simulink model "Full H-bridge motor driver simulator"  (R2018a)
settings: Solver=VariableStepAuto  StartTime=0.0  StopTime=20  RelTol=1e-3
undefined symbols (not defined in the file or in its folder): sigbuilder_block
libraries: fl_lib x12, nesl_utility x6, powerlib_meascontrol x1
settings Model: Creator=Kalindi  LastModifiedBy=Kalindi

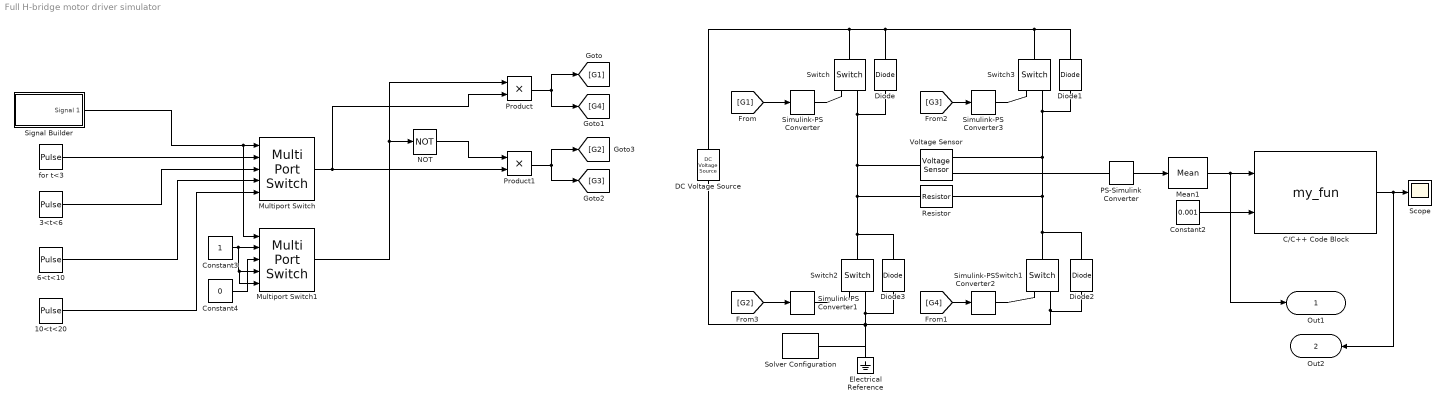
== system Full H-bridge motor driver simulator ==
  10<t<20 : DiscretePulseGenerator  PulseType=Time based  Amplitude=10  Period=0.03125  PulseWidth=79.392
  3<t<6 : DiscretePulseGenerator  PulseType=Time based  Amplitude=10  Period=0.03125  PulseWidth=49.386
  6<t<10 : DiscretePulseGenerator  PulseType=Time based  Amplitude=10  Period=0.03125  PulseWidth=19.956
  C/C++ Code Block : S-Function  InitFcn=try, set_param(gcb,'FunctionName','my_fun'), end  FunctionName=my_fun  Parameters=4.67,0.3234,0.4953  SFunctionModules=my_fun_wrapper  SFunctionDeploymentMode=off  EnableBusSupport=off  mask(S-Function Builder){R=0}
      mask help: Simulink:masks:SFunctionBuilder_MD
      mask init:
      | val = [[.9  0.75 0.75 1 1 .9 .9 1]',[1 1 0.75 0.75 .9 .9 1 .9]'];try , sys = get_param(gcb,'SfunBuilderFcnName');if isempty(sys), sys = get_param(gcb,'FunctionName'); end,catch, sys = get_param(gcb,'FunctionName'); end
      settings: CopyFcn=set_param(gcbh,'LinkStatus','none')  PreSaveFcn=try, set_param(gcb,'FunctionName','my_fun'), end  OpenFcn=sfunctionwizard(gcbh)
      mask Display: plot(val(:,1),val(:,2)),disp(sys), port_label('input',1,'Voltage'), port_label('input',2,'Torque'), port_label('output',1,'Speed')
  Constant2 : Constant  Value=0.001
  Constant3 : Constant
  Constant4 : Constant  Value=0
  DC Voltage Source : fl_lib/Electrical/Electrical Sources/DC Voltage Source  v0=10 V
  Diode{,1..3} (4 alike) : fl_lib/Electrical/Electrical Elements/Diode  Vf=0.6 V  Ron=0.3 Ohm  Goff=1e-8 1/Ohm  i_specify=off  i_priority=None  i=0 A  i_nominal_specify=off  i_nominal_unit=A  i_nominal_value=1  v_specify=off  v_priority=None  v=0 V  v_nominal_specify=off  v_nominal_unit=V  v_nominal_value=1
  Electrical Reference : fl_lib/Electrical/Electrical Elements/Electrical Reference
  Mean1 : powerlib_meascontrol/Measurements/Mean  Freq=32  Vinit=0  Ts=0
  Multiport Switch : MultiPortSwitch  Inputs=4
  Multiport Switch1 : MultiPortSwitch  Inputs=4
  NOT : Logic  Operator=NOT  IconShape=distinctive  AllPortsSameDT=off  OutDataTypeStr=boolean
  PS-Simulink Converter : nesl_utility/PS-Simulink Converter  PhysicalDomain=network_engine_domain  SubClassName=ps_output  LeftPortType=input  RightPortType=output  PseudoPeriodic=off  Frequencies=[]  Unit=V  AffineConversion=off
  Product : Product
  Product1 : Product
  Resistor : fl_lib/Electrical/Electrical Elements/Resistor  R=4 Ohm  i_specify=off  i_priority=None  i=0 A  i_nominal_specify=off  i_nominal_unit=A  i_nominal_value=1  v_specify=off  v_priority=None  v=0 V  v_nominal_specify=off  v_nominal_unit=V  v_nominal_value=1
  Scope : Scope
  Signal Builder : Subsystem  Tag=STV Subsys  LoadFcn=sigbuilder_block('load');  StartFcn=sigbuilder_block('start');  StopFcn=sigbuilder_block('stop');  ClipboardFcn=sigbuilder_block('clipboard');  mask(Sigbuilder block){tuvar=[0:10]}
      mask help: Simulink:masks:SigbuilderBlock_MD
      mask init:
      | if ~strcmp(get_param(bdroot(gcbh),'SimulationStatus'),'stopped') tuvar = sigbuilder_block('maskInit'); end
      settings: CopyFcn=sigbuilder_block('copy');  DeleteFcn=sigbuilder_block('delete');  ModelCloseFcn=sigbuilder_block('modelClose');  PreSaveFcn=sigbuilder_block('preSave');  PauseFcn=sigbuilder_block('pause');  ContinueFcn=sigbuilder_block('continue');  NameChangeFcn=sigbuilder_block('namechange');  OpenFcn=sigbuilder_block('open',[449.4 106.8 550.8 400.2 ]);  CloseFcn=sigbuilder_block('close');
      mask Display: plot(0, 0, 100, 100,[2, 2, 32, 32, 2], [68, 8, 8, 68, 68],[32, 2], [38, 38], [32, 19, 2],[53, 60, 44], [32, 17, 17, 2],[16, 16, 31, 31]);txt = getActiveGroup(gcbh);text(2, 100, txt,'verticalAlignment', 'top');
  Simulink-PS Converter{,1..3} (4 alike) : nesl_utility/Simulink-PS Converter  PhysicalDomain=network_engine_domain  SubClassName=ps_input  LeftPortType=input  RightPortType=output  PseudoPeriodic=off  Frequencies=[]  NoiseDistribution=none  NoiseParameters=[]  Unit=1  AffineConversion=off  FilteringAndDerivatives=provide  SimscapeFilterOrder=1  InputFilterTimeConstant=0.001  UdotUserProvided=0
  Solver Configuration : nesl_utility/Solver Configuration  PhysicalDomain=network_engine_domain  SubClassName=solver  LeftPortType=input  RightPortType=generic  Tones=[]  Harmonics=[]  SimulateNoise=off  Profile=off  UseLocalSampling=off  EnableSwitchedLinearOptims=on  FrequencyDomain=off  UseCCode=off  RelTol=0.001  AbsTol=1e-06  MinStep=1e-09  ToWorkspace=off  RevertToSquareIcSolve=off  NumHomotopyIterations=100  PhasorMode=off  PhasorModeNumHarmonics=1  DoDC=off  ResidualTolerance=1e-09  UseLocalSolver=on  LocalSolverChoice=NE_BACKWARD_EULER_ADVANCER  LocalSolverSampleTime=0.001  DoFixedCost=on  MaxNonlinIter=3  MaxModeIter=2  LinearAlgebra=Sparse  EquationFormulation=NE_TIME_EF  DelaysMemoryBudget=1024  AutomaticFiltering=on  FilteringTimeConstant=0.001
  Switch : fl_lib/Electrical/Electrical Elements/Switch  R_closed=.1e-11 Ohm  G_open=1e-8 1/Ohm  Threshold=0  i_specify=off  i_priority=None  i=0 A  i_nominal_specify=off  i_nominal_unit=A  i_nominal_value=1  v_specify=off  v_priority=None  v=0 V  v_nominal_specify=off  v_nominal_unit=V  v_nominal_value=1
      settings: SourceProductName=Simscape
  Switch1 : fl_lib/Electrical/Electrical Elements/Switch  R_closed=.1e-11 Ohm  G_open=1e-08 1/Ohm  Threshold=0  i_specify=off  i_priority=None  i=0 A  i_nominal_specify=off  i_nominal_unit=A  i_nominal_value=1  v_specify=off  v_priority=None  v=0 V  v_nominal_specify=off  v_nominal_unit=V  v_nominal_value=1
      settings: SourceProductName=Simscape
  Switch2 : fl_lib/Electrical/Electrical Elements/Switch  R_closed=.1e-11 Ohm  G_open=1e-08 1/Ohm  Threshold=0  i_specify=off  i_priority=None  i=0 A  i_nominal_specify=off  i_nominal_unit=A  i_nominal_value=1  v_specify=off  v_priority=None  v=0 V  v_nominal_specify=off  v_nominal_unit=V  v_nominal_value=1
      settings: SourceProductName=Simscape
  Switch3 : fl_lib/Electrical/Electrical Elements/Switch  R_closed=.1e-11 Ohm  G_open=1e-08 1/Ohm  Threshold=0  i_specify=off  i_priority=None  i=0 A  i_nominal_specify=off  i_nominal_unit=A  i_nominal_value=1  v_specify=off  v_priority=None  v=0 V  v_nominal_specify=off  v_nominal_unit=V  v_nominal_value=1
      settings: SourceProductName=Simscape
  Voltage Sensor : fl_lib/Electrical/Electrical Sensors/Voltage Sensor
  for t<3 : DiscretePulseGenerator  PulseType=Time based  Amplitude=10  Period=0.03125  PulseWidth=59.58
  Out1 : Outport  SignalName=Voltage
  Out2 : Outport  Port=2  SignalName=w
  wires:
  Multiport Switch1/1 -> Product/1, NOT/1
  Multiport Switch/1 -> Product/2, Product1/2
  Product/1 -> [G1], [G4]
  Product1/1 -> [G3], [G2]
  NOT/1 -> Product1/1
  Mean1/1 -> Out1/1, C/C++ Code Block/1
  [G2] -> Simulink-PS Converter1/1
  [G3] -> Simulink-PS Converter3/1
  [G4] -> Simulink-PS Converter2/1
  [G1] -> Simulink-PS Converter/1
  Constant2/1 -> C/C++ Code Block/2
  C/C++ Code Block/1 -> Out2/1, Scope/1
  Constant3/1 -> Multiport Switch1/5, Multiport Switch1/4, Multiport Switch1/2
  Signal Builder/1(Signal 1) -> Multiport Switch1/1, Multiport Switch/1
  Constant4/1 -> Multiport Switch1/3
  6<t<10/1 -> Multiport Switch/4
  3<t<6/1 -> Multiport Switch/3
  10<t<20/1 -> Multiport Switch/5
  for t<3/1 -> Multiport Switch/2
  PS-Simulink Converter/1 -> Mean1/1
  connections:
  Switch3/RConn2 -- Diode1/LConn1 -- Voltage Sensor/RConn2 -- Resistor/RConn1 -- Diode2/RConn1 -- Switch1/LConn1
  Simulink-PS Converter3/RConn1 -- Switch3/RConn1
  Simulink-PS Converter2/RConn1 -- Switch1/RConn1
  Simulink-PS Converter1/RConn1 -- Switch2/RConn1
  Simulink-PS Converter/RConn1 -- Switch/RConn1
  Switch/LConn1 -- Switch3/LConn1 -- Diode1/RConn1 -- Diode/RConn1 -- DC Voltage Source/LConn1
  Switch/RConn2 -- Diode/LConn1 -- Voltage Sensor/LConn1 -- Resistor/LConn1 -- Diode3/RConn1 -- Switch2/LConn1
  Switch2/RConn2 -- Diode3/LConn1 -- Solver Configuration/RConn1 -- Electrical Reference/LConn1 -- Diode2/LConn1 -- Switch1/RConn2 -- DC Voltage Source/RConn1
  PS-Simulink Converter/LConn1 -- Voltage Sensor/RConn1

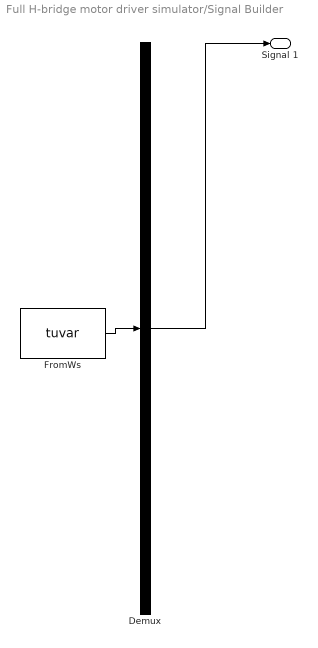
== system Full H-bridge motor driver simulator/Signal Builder ==
  Demux : Demux  Tag=STV Demux  Outputs=1
  FromWs : FromWorkspace  Tag=STV FromWs  VariableName=tuvar  SampleTime=0
      SigBuilderData=|
      | common.afterFinalStr = 'Extrapolate'
      | common.sampleTime = 0
      | dataSet.timeRange = [0 20]
      | dataSet.name = 'Group 1'
      | sbobj.Groups.Name = 'Group 1'
      | sbobj.Groups.Signals.Name = 'Signal 1'
      | sbobj.Groups.Signals.XData = [0 3 3 6 6 10 10 20]
      | sbobj.Groups.Signals.YData = [1 1 2 2 3 3 4 4]
      | sbobj.Groups.TimeRange = [0 20]
  Signal 1 : Outport  Tag=STV Outport
  wires:
  Demux/1 -> Signal 1/1
  FromWs/1 -> Demux/1
